simulink subsystem "environment"  (R2024b)
settings: Solver=VariableStepAuto  StartTime=0.0  StopTime=10.0  RelTol=1e-3
settings Model: Creator=yagiz  LastModifiedBy=yagiz

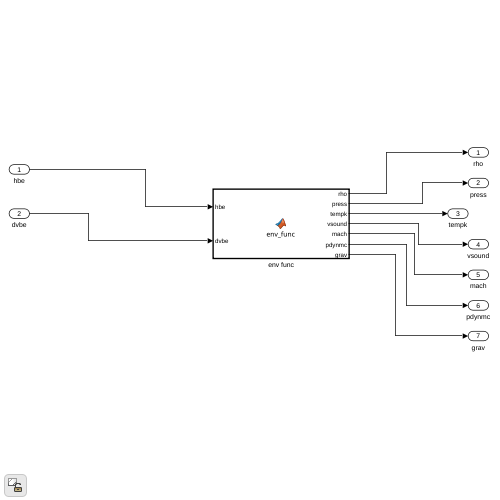
[thumbnail: Simulink's stored preview of the top-level diagram]
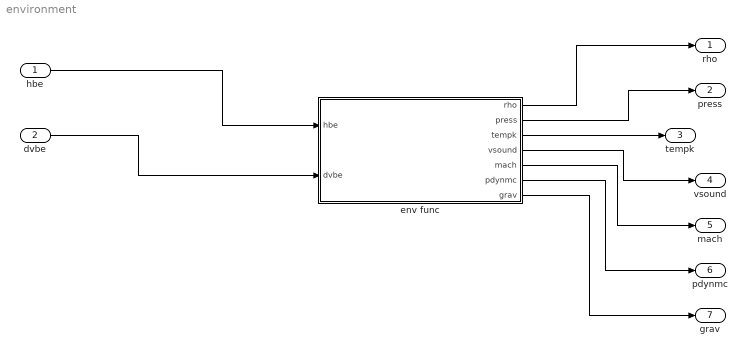
== system environment ==
  hbe : Inport
  dvbe : Inport  Port=2
  env func : MATLAB Function  TreatAsAtomicUnit=on
  rho : Outport
  press : Outport  Port=2
  tempk : Outport  Port=3
  vsound : Outport  Port=4
  mach : Outport  Port=5
  pdynmc : Outport  Port=6
  grav : Outport  Port=7
  wires:
  hbe/1 -> env func/1(hbe)
  dvbe/1 -> env func/2(dvbe)
  env func/1(rho) -> rho/1
  env func/2(press) -> press/1
  env func/3(tempk) -> tempk/1
  env func/4(vsound) -> vsound/1
  env func/5(mach) -> mach/1
  env func/6(pdynmc) -> pdynmc/1
  env func/7(grav) -> grav/1

== matlab function environment/env func ==
  data: hbe input; rho output; dvbe input; press output; tempk output; vsound output; mach output; pdynmc output; grav output
function [rho, press, tempk, vsound, mach, pdynmc, grav] = env_func(hbe, dvbe)

R_AIR = 287.058;
G0    = 9.80665;
REARTH     = 6.3781e6;
G_CONST    = 6.674e-11;
EARTH_MASS = 5.9722e24;

h = max(hbe, 0.0);

if h <= 11000.0
    T = 288.15 - 6.5e-3 * h;
    P = 101325.0 * (T / 288.15)^5.25588;
elseif h <= 20000.0
    T = 216.65;
    P = 22632.1 * exp(-G0 / (R_AIR * T) * (h - 11000.0));
elseif h <= 32000.0
    T = 216.65 + 1.0e-3 * (h - 20000.0);
    P = 5474.89 * (T / 216.65)^(-G0 / (R_AIR * 1.0e-3));
else
    T = 228.65 + 2.8e-3 * (h - 32000.0);
    P = 868.019 * (T / 228.65)^(-G0 / (R_AIR * 2.8e-3));
end

rho    = P / (R_AIR * T);
press  = P;
tempk  = T;
vsound = sqrt(1.4 * R_AIR * T);
mach   = abs(dvbe / vsound);
pdynmc = 0.5 * rho * dvbe * dvbe;
rad    = REARTH + h;
grav   = G_CONST * EARTH_MASS / (rad * rad);
function y = fcn(u)

y = u;
